simulink model "train_control"  (R2014b)
settings: Solver=FixedStepDiscrete  StartTime=0.0  StopTime=100000  FixedStep=0.01  MaxStep=0.0001  RelTol=1e-3
settings Model: Creator=sand080  LastModifiedBy=sand080
settings DataIOCC: LimitDataPoints=off

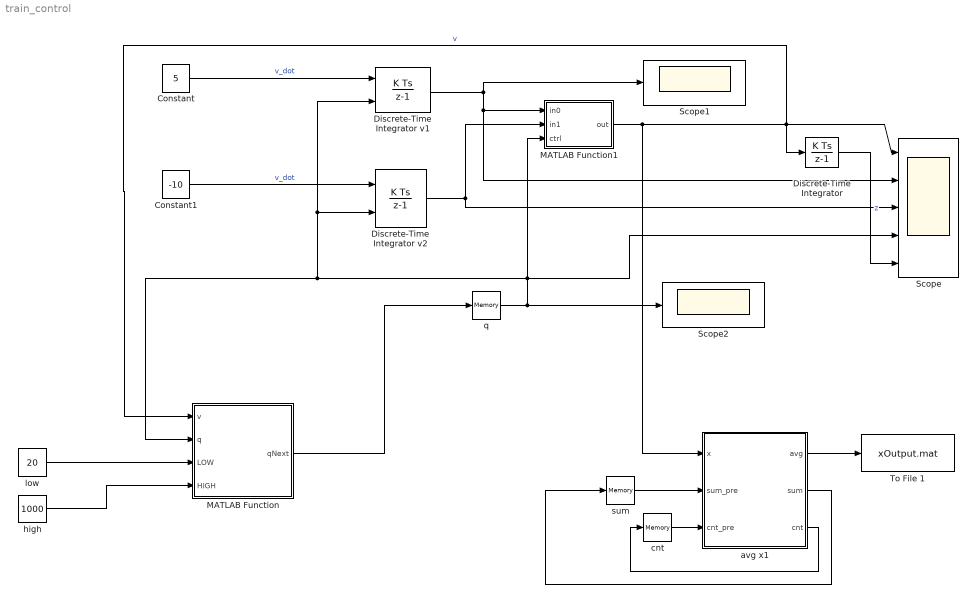
== system train_control ==
  Constant : Constant  Value=5
  Constant1 : Constant  Priority=1  Value=-10
  Discrete-Time Integrator : DiscreteIntegrator  InitialConditionSetting=State (most efficient)  SampleTime=-1
  Discrete-Time Integrator v1 : DiscreteIntegrator  ExternalReset=either  InitialCondition=20  InitialConditionSetting=State (most efficient)  SampleTime=-1
  Discrete-Time Integrator v2 : DiscreteIntegrator  ExternalReset=either  InitialCondition=1000  InitialConditionSetting=State (most efficient)  SampleTime=-1
  MATLAB Function : MATLAB Function  Priority=1  TreatAsAtomicUnit=on
  MATLAB Function1 : MATLAB Function  TreatAsAtomicUnit=on
  Scope : Scope  NumInputPorts=5
      settings: TickLabels=on  ShowLegends=on  YMin=0~0~-1000~0~0  YMax=1500~1500~1000~1~1.5e+07
  Scope1 : Scope
  Scope2 : Scope
      settings: SaveName=ScopeData2
  To File 1 : ToFile  Filename=xOutput.mat
      settings: Decimation=10000000
  avg x1 : MATLAB Function  Priority=4  TreatAsAtomicUnit=on
  cnt : Memory
  high : Constant  Value=1000
  low : Constant  Value=20
  q : Memory
  sum : Memory
  wires:
  MATLAB Function/1(qNext) -> q/1
  avg x1/2(sum) -> sum/1
  avg x1/3(cnt) -> cnt/1
  cnt/1 -> avg x1/3(cnt_pre)
  sum/1 -> avg x1/2(sum_pre)
  avg x1/1(avg) -> To File 1/1
  Constant/1 -> Discrete-Time Integrator v1/1  "v_dot"
  Discrete-Time Integrator v2/1 -> MATLAB Function1/2(in1), Scope/3
  Constant1/1 -> Discrete-Time Integrator v2/1  "v_dot"
  Discrete-Time Integrator v1/1 -> Scope/2, MATLAB Function1/1(in0), Scope1/1
  MATLAB Function1/1(out) -> avg x1/1(x), Discrete-Time Integrator/1, Scope/1, MATLAB Function/1(v)  "v"
  low/1 -> MATLAB Function/3(LOW)
  high/1 -> MATLAB Function/4(HIGH)
  Discrete-Time Integrator/1 -> Scope/5  "z"
  q/1 -> Scope2/1, Scope/4, MATLAB Function1/3(ctrl), Discrete-Time Integrator v1/2, Discrete-Time Integrator v2/2, MATLAB Function/2(q)

== matlab function train_control/MATLAB Function1 ==
  data: in0 input; in1 input; ctrl input; out output
function out = select(in0,in1,ctrl)
%#codegen
if(ctrl==0)
    out=in0;
else
    out=in1;
end

== matlab function train_control/MATLAB Function ==
  data: v input; q input; qNext output; LOW input; HIGH input
function qNext = phi(v,q, LOW, HIGH)
%#codegen
if q==0 && v < HIGH
    qNext=0;
elseif q==0 && v >= HIGH
    qNext=1;
elseif q==1 && v > LOW
    qNext=1;
elseif q==1 && v <= LOW
    qNext=0;
else
    qNext=-1; %this should never execute
end

== matlab function train_control/avg x1 ==
  data: x input; avg output; sum output; cnt output; sum_pre input; cnt_pre input
function [avg, sum,cnt] = fcn(x,  sum_pre, cnt_pre)
%#codegen

cnt=cnt_pre+1;
sum=sum_pre+x;
avg=sum/cnt;
